simulink model "generacjaSygnalu"  (R2015a)
settings: Solver=ode4  StartTime=0.0  StopTime=simulationTime  FixedStep=sampleTime  RelTol=1e-3
values from neighbouring files (symbols this model uses):
  DEN = zeros(length(h_n), 6)    [model_strejc2.m]    (also in uruchom_symulacja_szumy.m = sym2poly((s+1)*(2*s+1)*(3*s+1)*(4*s+1)*(5*s+1)*(6*s+1)))
  NUM = 1    [model_strejc2.m]    (also in uruchom_symulacja_szumy.m)
  sampleTime = 0.01    [uruchom_symulacja_szumy.m]
libraries: simulink x1
settings Model: Creator=Kamil  LastModifiedBy=Kamil

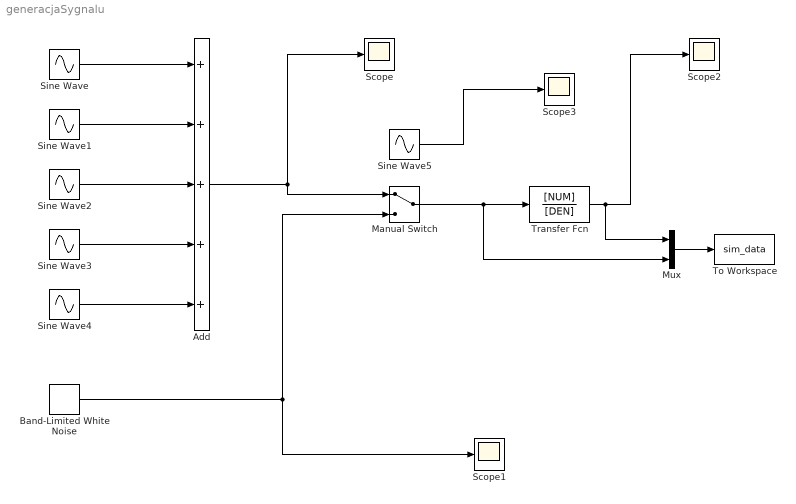
== system generacjaSygnalu ==
  Add : Sum  Inputs=+++++
  Band-Limited White Noise : simulink/Sources/Band-Limited White Noise  Cov=[0.0001]  Ts=sampleTime  seed=[23341]
  Manual Switch : ManualSwitch
  Mux : Mux  Inputs=2
  Scope{,1..3} (4 alike) : Scope
      Scope2 settings: TimeRange=150  YMin=-0.004  YMax=0.005000000000000001  SaveName=ScopeData2
      Scope3 settings: SaveName=ScopeData3
  Sine Wave : Sin  Amplitude=5  Frequency=0.05  SampleTime=0
  Sine Wave1 : Sin  Amplitude=2  Frequency=0.5  Phase=pi  SampleTime=0
  Sine Wave2 : Sin  Amplitude=2  Frequency=3  SampleTime=0
  Sine Wave3 : Sin  Amplitude=15  Frequency=0.01  Phase=pi/2  SampleTime=0
  Sine Wave4 : Sin  Amplitude=15  Frequency=5  SampleTime=0
  Sine Wave5 : Sin  Amplitude=0.5  Bias=0.02  Frequency=10  SampleTime=0
  To Workspace : ToWorkspace  VariableName=sim_data  SaveFormat=Structure With Time  SampleTime=-1
  Transfer Fcn : TransferFcn  Numerator=[NUM]  Denominator=[DEN]
  wires:
  Sine Wave4/1 -> Add/5
  Sine Wave3/1 -> Add/4
  Sine Wave2/1 -> Add/3
  Sine Wave1/1 -> Add/2
  Sine Wave/1 -> Add/1
  Add/1 -> Manual Switch/1, Scope/1
  Band-Limited White Noise/1 -> Manual Switch/2, Scope1/1
  Transfer Fcn/1 -> Mux/1, Scope2/1
  Mux/1 -> To Workspace/1
  Sine Wave5/1 -> Scope3/1
  Manual Switch/1 -> Mux/2, Transfer Fcn/1
